simulink model "CS637Assignment3_2_2"  (R2022a)
settings: Solver=FixedStepAuto  StartTime=0.0  StopTime=1000.0  RelTol=1e-3
model workspace (MAT data in the model file):
  A = Simulink.Parameter
  A.Value = [0  1; 0  0]
  A.DataType = 'custom_type_1'
  A.Complexity = 'real'
  A.Dimensions = [2 2]
  B = Simulink.Parameter
  B.Value = [0.4; 1]
  B.DataType = 'custom_type_1'
  B.Complexity = 'real'
  B.Dimensions = [2 1]
  C = Simulink.Parameter
  C.Value = [1 0]
  C.DataType = 'custom_type_1'
  C.Complexity = 'real'
  C.Dimensions = [1 2]
  Kr = Simulink.Parameter
  Kr.Value = 1
  Kr.DataType = 'custom_type_1'
  Kr.Complexity = 'real'
  Kr.Dimensions = [1 1]
  L = Simulink.Parameter
  L.Value = [6; 5]
  L.DataType = 'custom_type_1'
  L.Complexity = 'real'
  L.Dimensions = [2 1]
  k1 = Simulink.Parameter
  k1.Value = 1
  k1.DataType = 'custom_type_1'
  k1.Complexity = 'real'
  k1.Dimensions = [1 1]
  k2 = Simulink.Parameter
  k2.Value = 1.6
  k2.DataType = 'custom_type_1'
  k2.Complexity = 'real'
  k2.Dimensions = [1 1]
settings Model: Creator=kaush  LastModifiedBy=kaush
settings OptimizationCC: OptimizeBlockIOStorage=off  ZeroExternalMemoryAtStartup=off  ZeroInternalMemoryAtStartup=off  OptimizeDataStoreBuffers=off  BusAssignmentInplaceUpdate=off
settings DebuggingCC: SFUnexpectedBacktrackingDiag=warning  SFNoUnconditionalDefaultTransitionDiag=warning
settings RTWCC: GenCodeOnly=on  GenerateReport=on  Toolchain=MinGW64 | gmake (64-bit Windows)  BuildConfiguration=Debug  LaunchReport=on  TargetLang=C++
settings CodeAppCC: ForceParamTrailComments=on  MATLABSourceComments=on  EnableCustomComments=on
settings GRTTargetCC: TargetLangStandard=C++11 (ISO)  CombineSignalStateStructs=on  CodeInterfacePackaging=C++ class  SupportVariableSizeSignals=on  MultiInstanceErrorCode=Warning

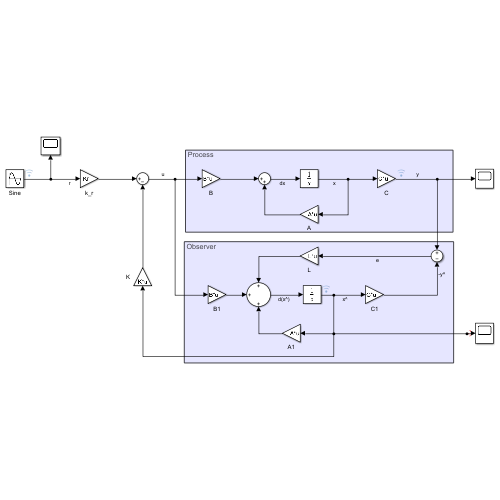
[thumbnail: Simulink's stored preview of the top-level diagram]
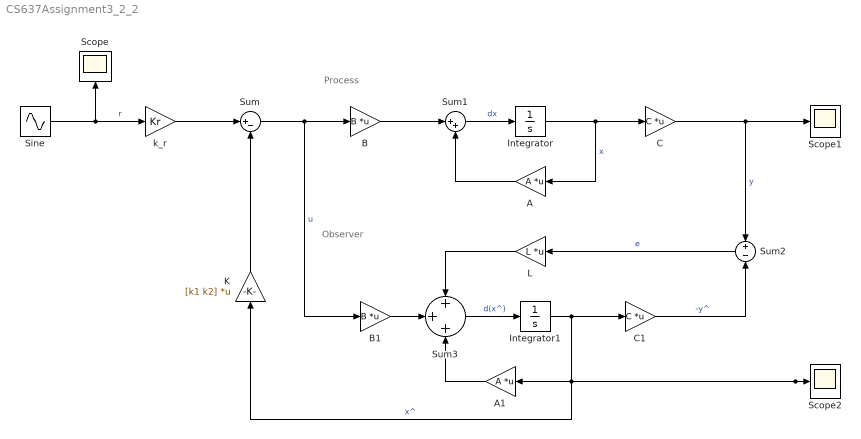
== system CS637Assignment3_2_2 ==
  note: Process
  note: Observer
  A : Gain  Gain=A  Multiplication=Matrix(K*u)
  A1 : Gain  Gain=A  Multiplication=Matrix(K*u)
  B : Gain  Gain=B  Multiplication=Matrix(K*u)
  B1 : Gain  Gain=B  Multiplication=Matrix(K*u)
  C : Gain  Gain=C  Multiplication=Matrix(K*u)
  C1 : Gain  Gain=C  Multiplication=Matrix(K*u)
  Integrator : Integrator
  Integrator1 : Integrator
  K : Gain  Gain=[k1 k2]  Multiplication=Matrix(K*u)
  L : Gain  Gain=L  Multiplication=Matrix(K*u)
  Scope : Scope
  Scope1 : Scope
  Scope2 : Scope
  Sine : Sin  SampleTime=0
  Sum : Sum  Inputs=|+-
  Sum1 : Sum  Inputs=|++
  Sum2 : Sum  Inputs=+-
  Sum3 : Sum  Inputs=+++
  k_r : Gain  Gain=Kr
  wires:
  Sine/1 -> k_r/1, Scope/1  "r"
  k_r/1 -> Sum/1
  Sum/1 -> B1/1, B/1  "u"
  B/1 -> Sum1/1
  Sum1/1 -> Integrator/1  "dx"
  A/1 -> Sum1/2
  Integrator/1 -> A/1, C/1  "x"
  C/1 -> Scope1/1, Sum2/1  "y"
  B1/1 -> Sum3/2
  Sum2/1 -> L/1  "e"
  Sum3/1 -> Integrator1/1  "d(x^)"
  A1/1 -> Sum3/3
  C1/1 -> Sum2/2  "-y^"
  Integrator1/1 -> Scope2/1, K/1, A1/1, C1/1  "x^"
  L/1 -> Sum3/1
  K/1 -> Sum/2
